simulink model "QuarterBusActiveSuspensionModel"  (R2025b)
settings: Solver=ode23t  StartTime=0.0  StopTime=10  RelTol=1e-3
undefined symbols (not defined in the file): b1, b2, k1, k2, kd, ki, kp, m1, m2, SP
settings Model: Creator=kanch  LastModifiedBy=kanch
settings DataIOCC: ExternalInput=inputDataStructure  LoadExternalInput=on

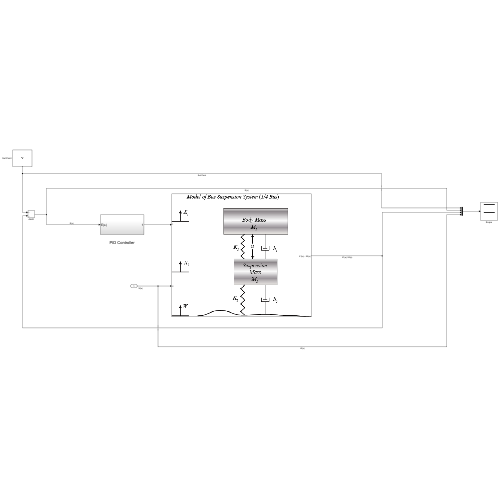
[thumbnail: Simulink's stored preview of the top-level diagram]
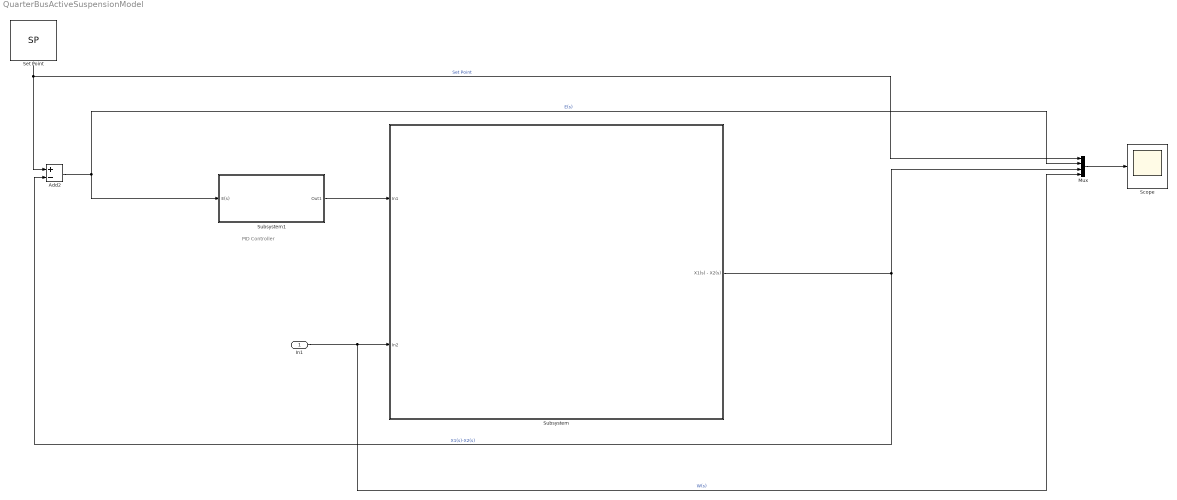
== system QuarterBusActiveSuspensionModel ==
  note: PID Controller
  In1 : Inport
  Add2 : Sum  Inputs=+-
  Mux : Mux
  Scope : Scope
      settings: ActiveDisplayYMinimum=-0.027667801865854394  ActiveDisplayYMaximum=0.028257502423467348  DataLoggingVariableName=Scope_Data
  Set Point : Constant  Value=SP
  Subsystem : Subsystem
      mask Display: image('susp1.png');
  Subsystem1 : Subsystem
  wires:
  Add2/1 -> Subsystem1/1(E(s)), Mux/2  "E(s)"
  Mux/1 -> Scope/1
  Set Point/1 -> Add2/1, Mux/1  "Set Point"
  Subsystem/1(X1(s) - X2(s)) -> Add2/2, Mux/3  "X1(s)-X2(s)"
  In1/1 -> Mux/4, Subsystem/2(In2)  "W(s)"
  Subsystem1/1(Out1) -> Subsystem/1(In1)

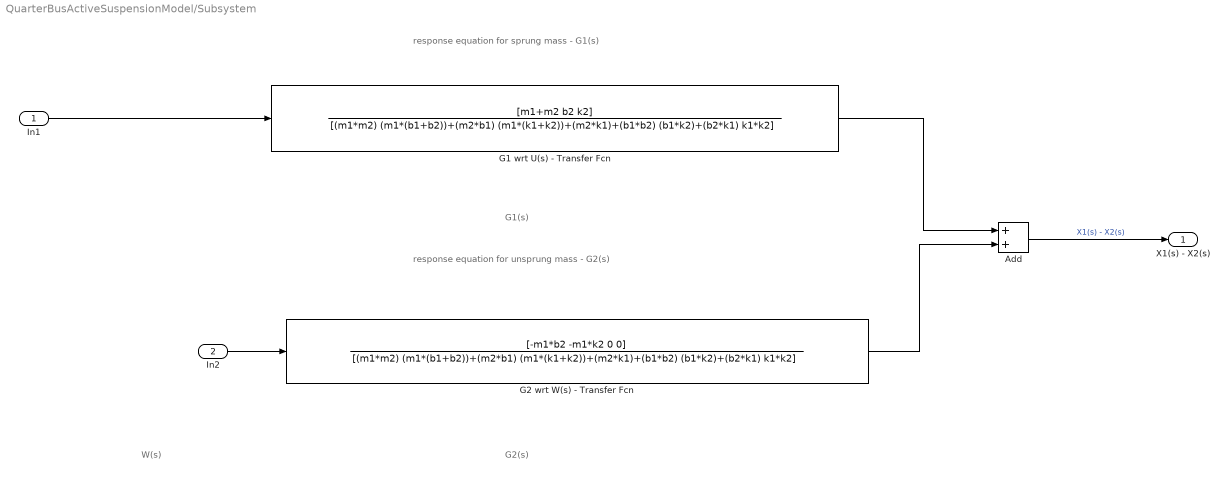
== system QuarterBusActiveSuspensionModel/Subsystem ==
  note: G2(s)
  note: W(s)
  note: response equation for sprung mass - G1(s)
  note: response equation for unsprung mass - G2(s)
  note: G1(s)
  In1 : Inport
  In2 : Inport  Port=2
  Add : Sum
  G1 wrt U(s) - Transfer Fcn : TransferFcn  Numerator=[m1+m2 b2 k2]  Denominator=[(m1*m2) (m1*(b1+b2))+(m2*b1) (m1*(k1+k2))+(m2*k1)+(b1*b2) (b1*k2)+(b2*k1) k1*k2]
  G2 wrt W(s) - Transfer Fcn : TransferFcn  Numerator=[-m1*b2 -m1*k2 0 0]  Denominator=[(m1*m2) (m1*(b1+b2))+(m2*b1) (m1*(k1+k2))+(m2*k1)+(b1*b2) (b1*k2)+(b2*k1) k1*k2]
  X1(s) - X2(s) : Outport
  wires:
  G2 wrt W(s) - Transfer Fcn/1 -> Add/2
  In1/1 -> G1 wrt U(s) - Transfer Fcn/1
  G1 wrt U(s) - Transfer Fcn/1 -> Add/1
  In2/1 -> G2 wrt W(s) - Transfer Fcn/1
  Add/1 -> X1(s) - X2(s)/1  "X1(s) - X2(s)"

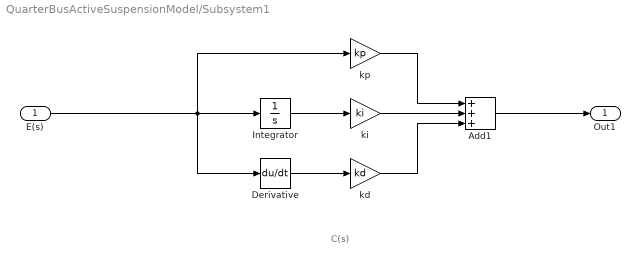
== system QuarterBusActiveSuspensionModel/Subsystem1 ==
  note: C(s)
  E(s) : Inport
  Add1 : Sum  Inputs=+++
  Derivative : Derivative
  Integrator : Integrator
  kd : Gain  Gain=kd
  ki : Gain  Gain=ki
  kp : Gain  Gain=kp
  Out1 : Outport
  wires:
  Derivative/1 -> kd/1
  E(s)/1 -> Derivative/1, kp/1, Integrator/1
  Add1/1 -> Out1/1
  ki/1 -> Add1/2
  kp/1 -> Add1/1
  Integrator/1 -> ki/1
  kd/1 -> Add1/3
